simulink model "sim_OKID_open_loop"  (R2014b)
settings: Solver=ode45  StartTime=0.0  StopTime=10.0  RelTol=1e-3
values from neighbouring files (symbols this model uses):
  A = zp2ss(2, P ,8)    [OKID_closed_loop.m]
  B = H    [OKID_closed_loop.m]    (also in OKID_fun_WT02_6.m = Btemp(:, 1:r))
  C = [-4.268707812 5.80698373674 2.29894982459 -1.81972727507 -0.693726564507 -1.15322974081 0.496155860115 0.368426779263]    [OKIDData.mat]
  Ts = 1800    [OKIDData.mat]    (also in OKID_closed_loop.m = 0.005)
settings Model: Creator=123  LastModifiedBy=123

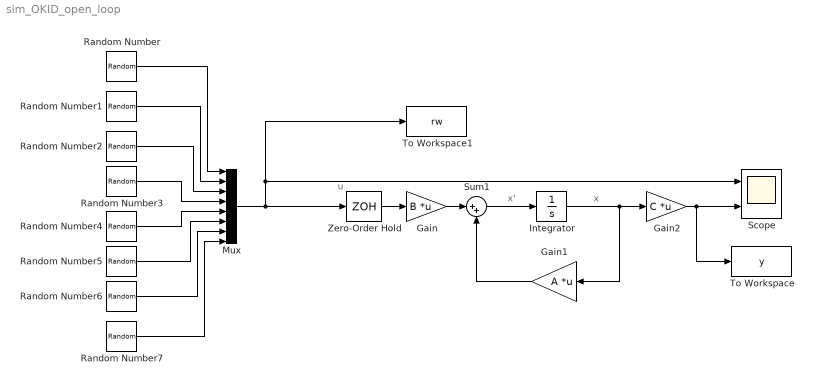
== system sim_OKID_open_loop ==
  note: u
  note: x'
  note: x
  Gain : Gain  Gain=B  Multiplication=Matrix(K*u)
  Gain1 : Gain  Gain=A  Multiplication=Matrix(K*u)
  Gain2 : Gain  Gain=C  Multiplication=Matrix(K*u)
  Integrator : Integrator
  Mux : Mux  Inputs=8
  Random Number : RandomNumber  SampleTime=Ts
  Random Number1 : RandomNumber  Seed=1  SampleTime=Ts
  Random Number2 : RandomNumber  Seed=2  SampleTime=Ts
  Random Number3 : RandomNumber  Seed=3  SampleTime=Ts
  Random Number4 : RandomNumber  Seed=4  SampleTime=Ts
  Random Number5 : RandomNumber  Seed=5  SampleTime=Ts
  Random Number6 : RandomNumber  Seed=6  SampleTime=Ts
  Random Number7 : RandomNumber  Seed=7  SampleTime=Ts
  Scope : Scope  NumInputPorts=2
      settings: YMin=-5~-5  YMax=5~5
  Sum1 : Sum  Inputs=|++
  To Workspace : ToWorkspace  VariableName=y  SampleTime=-1
  To Workspace1 : ToWorkspace  VariableName=rw  SampleTime=-1
  Zero-Order Hold : ZeroOrderHold  SampleTime=Ts
  wires:
  Integrator/1 -> Gain1/1, Gain2/1
  Mux/1 -> Zero-Order Hold/1, To Workspace1/1, Scope/1
  Sum1/1 -> Integrator/1
  Gain/1 -> Sum1/1
  Gain1/1 -> Sum1/2
  Gain2/1 -> To Workspace/1, Scope/2
  Zero-Order Hold/1 -> Gain/1
  Random Number/1 -> Mux/1
  Random Number1/1 -> Mux/2
  Random Number2/1 -> Mux/3
  Random Number3/1 -> Mux/4
  Random Number4/1 -> Mux/5
  Random Number5/1 -> Mux/6
  Random Number6/1 -> Mux/7
  Random Number7/1 -> Mux/8
